simulink model "VCU_CS75_9_30"  (R2014a)
settings: Solver=FixedStepDiscrete  StartTime=0.0  StopTime=25  FixedStep=0.0005  RelTol=1e-3
undefined symbols (not defined in the file or in its folder): APAStatus_2D4, ecucoder_acal, I_SW01_L, LDW, ST_comd, TX2D4
libraries: simulink x881, ec5744lib x37
(part 13 of 30)

== system VCU_CS75_9_30/长安CS75底盘程序，20ms一次/BSW_Input/DBC转化的messages（存底）/ReceiveMessages12/HU_LASSetting_0x541/HU_LDWShakeLev_Sub ==
  In1 : Inport
  Out1 : Outport
  wires:
  In1/1 -> Out1/1

== system VCU_CS75_9_30/长安CS75底盘程序，20ms一次/BSW_Input/DBC转化的messages（存底）/ReceiveMessages12/HU_LASSetting_0x541/HU_LdwSensitivity_Sub ==
  In1 : Inport
  Out1 : Outport
  wires:
  In1/1 -> Out1/1

== system VCU_CS75_9_30/长安CS75底盘程序，20ms一次/BSW_Input/DBC转化的messages（存底）/ReceiveMessages12/HU_LASSetting_0x541/HU_LockCtrlEnable_Sub ==
  In1 : Inport
  Out1 : Outport
  wires:
  In1/1 -> Out1/1

== system VCU_CS75_9_30/长安CS75底盘程序，20ms一次/BSW_Input/DBC转化的messages（存底）/ReceiveMessages12/HU_LASSetting_0x541/HU_ObstacleSafeDistanceSet_Sub ==
  In1 : Inport
  Out1 : Outport
  wires:
  In1/1 -> Out1/1

== system VCU_CS75_9_30/长安CS75底盘程序，20ms一次/BSW_Input/DBC转化的messages（存底）/ReceiveMessages12/HU_LASSetting_0x541/HU_OverspeedSoundWarEnable_Sub ==
  In1 : Inport
  Out1 : Outport
  wires:
  In1/1 -> Out1/1

== system VCU_CS75_9_30/长安CS75底盘程序，20ms一次/BSW_Input/DBC转化的messages（存底）/ReceiveMessages12/HU_LASSetting_0x541/HU_OverspeedWarningEnable_Sub ==
  In1 : Inport
  Out1 : Outport
  wires:
  In1/1 -> Out1/1

== system VCU_CS75_9_30/长安CS75底盘程序，20ms一次/BSW_Input/DBC转化的messages（存底）/ReceiveMessages12/HU_LASSetting_0x541/HU_OverspeedWarningOffset_Sub ==
  In1 : Inport
  Out1 : Outport
  wires:
  In1/1 -> Out1/1

== system VCU_CS75_9_30/长安CS75底盘程序，20ms一次/BSW_Input/DBC转化的messages（存底）/ReceiveMessages12/HU_LASSetting_0x541/HU_ParkingConfirm_Sub ==
  In1 : Inport
  Out1 : Outport
  wires:
  In1/1 -> Out1/1

== system VCU_CS75_9_30/长安CS75底盘程序，20ms一次/BSW_Input/DBC转化的messages（存底）/ReceiveMessages12/HU_LASSetting_0x541/HU_ParkingResume_Sub ==
  In1 : Inport
  Out1 : Outport
  wires:
  In1/1 -> Out1/1

== system VCU_CS75_9_30/长安CS75底盘程序，20ms一次/BSW_Input/DBC转化的messages（存底）/ReceiveMessages12/HU_LASSetting_0x541/HU_RCWEnable_Sub ==
  In1 : Inport
  Out1 : Outport
  wires:
  In1/1 -> Out1/1

== system VCU_CS75_9_30/长安CS75底盘程序，20ms一次/BSW_Input/DBC转化的messages（存底）/ReceiveMessages12/HU_LASSetting_0x541/HU_RCWSoundEnable_Sub ==
  In1 : Inport
  Out1 : Outport
  wires:
  In1/1 -> Out1/1

== system VCU_CS75_9_30/长安CS75底盘程序，20ms一次/BSW_Input/DBC转化的messages（存底）/ReceiveMessages12/HU_LASSetting_0x541/HU_RemoteDistanceSet_Sub ==
  In1 : Inport
  Out1 : Outport
  wires:
  In1/1 -> Out1/1

== system VCU_CS75_9_30/长安CS75底盘程序，20ms一次/BSW_Input/DBC转化的messages（存底）/ReceiveMessages12/HU_LASSetting_0x541/HU_SEWEnable_Sub ==
  In1 : Inport
  Out1 : Outport
  wires:
  In1/1 -> Out1/1

== system VCU_CS75_9_30/长安CS75底盘程序，20ms一次/BSW_Input/DBC转化的messages（存底）/ReceiveMessages12/HU_LASSetting_0x541/HU_SLASwitch_Sub ==
  In1 : Inport
  Out1 : Outport
  wires:
  In1/1 -> Out1/1

== system VCU_CS75_9_30/长安CS75底盘程序，20ms一次/BSW_Input/DBC转化的messages（存底）/ReceiveMessages12/HU_LASSetting_0x541/HU_Uls_BSD_Activation_Sub ==
  In1 : Inport
  Out1 : Outport
  wires:
  In1/1 -> Out1/1

== system VCU_CS75_9_30/长安CS75底盘程序，20ms一次/BSW_Input/DBC转化的messages（存底）/ReceiveMessages12/HU_LASSetting_0x541/HU_Uls_FKP_Activation_Sub ==
  In1 : Inport
  Out1 : Outport
  wires:
  In1/1 -> Out1/1

== system VCU_CS75_9_30/长安CS75底盘程序，20ms一次/BSW_Input/DBC转化的messages（存底）/ReceiveMessages13/SAS_108/SAS_CRCCheck_Sub ==
  In1 : Inport
  Out1 : Outport
  wires:
  In1/1 -> Out1/1

== system VCU_CS75_9_30/长安CS75底盘程序，20ms一次/BSW_Input/DBC转化的messages（存底）/ReceiveMessages13/SAS_108/SAS_Calibrated_Sub ==
  In1 : Inport
  Out1 : Outport
  wires:
  In1/1 -> Out1/1

== system VCU_CS75_9_30/长安CS75底盘程序，20ms一次/BSW_Input/DBC转化的messages（存底）/ReceiveMessages13/SAS_108/SAS_RollingCounter_Sub ==
  In1 : Inport
  Out1 : Outport
  wires:
  In1/1 -> Out1/1

== system VCU_CS75_9_30/长安CS75底盘程序，20ms一次/BSW_Input/DBC转化的messages（存底）/ReceiveMessages13/SAS_108/SAS_SASFailure_Sub ==
  In1 : Inport
  Out1 : Outport
  wires:
  In1/1 -> Out1/1

== system VCU_CS75_9_30/长安CS75底盘程序，20ms一次/BSW_Input/DBC转化的messages（存底）/ReceiveMessages13/SAS_108/SAS_SteeringAngleSpeed_Sub ==
  In1 : Inport
  Out1 : Outport
  wires:
  In1/1 -> Out1/1

== system VCU_CS75_9_30/长安CS75底盘程序，20ms一次/BSW_Input/DBC转化的messages（存底）/ReceiveMessages13/SAS_108/SAS_SteeringAngleValid_Sub ==
  In1 : Inport
  Out1 : Outport
  wires:
  In1/1 -> Out1/1

== system VCU_CS75_9_30/长安CS75底盘程序，20ms一次/BSW_Input/DBC转化的messages（存底）/ReceiveMessages13/SAS_108/SAS_SteeringAngle_Sub ==
  In1 : Inport
  Out1 : Outport
  wires:
  In1/1 -> Out1/1

== system VCU_CS75_9_30/长安CS75底盘程序，20ms一次/BSW_Input/DBC转化的messages（存底）/ReceiveMessages14/SCM_3B8/SCM_ACCCancel_Sub ==
  In1 : Inport
  Out1 : Outport
  wires:
  In1/1 -> Out1/1

== system VCU_CS75_9_30/长安CS75底盘程序，20ms一次/BSW_Input/DBC转化的messages（存底）/ReceiveMessages14/SCM_3B8/SCM_ACCOn_Sub ==
  In1 : Inport
  Out1 : Outport
  wires:
  In1/1 -> Out1/1

== system VCU_CS75_9_30/长安CS75底盘程序，20ms一次/BSW_Input/DBC转化的messages（存底）/ReceiveMessages14/SCM_3B8/SCM_IACCOn_Sub ==
  In1 : Inport
  Out1 : Outport
  wires:
  In1/1 -> Out1/1

== system VCU_CS75_9_30/长安CS75底盘程序，20ms一次/BSW_Input/DBC转化的messages（存底）/ReceiveMessages14/SCM_3B8/SCM_Resume_Sub ==
  In1 : Inport
  Out1 : Outport
  wires:
  In1/1 -> Out1/1

== system VCU_CS75_9_30/长安CS75底盘程序，20ms一次/BSW_Input/DBC转化的messages（存底）/ReceiveMessages14/SCM_3B8/SCM_Speeddecrease_Sub ==
  In1 : Inport
  Out1 : Outport
  wires:
  In1/1 -> Out1/1

== system VCU_CS75_9_30/长安CS75底盘程序，20ms一次/BSW_Input/DBC转化的messages（存底）/ReceiveMessages14/SCM_3B8/SCM_TimeGap_Sub ==
  In1 : Inport
  Out1 : Outport
  wires:
  In1/1 -> Out1/1

== system VCU_CS75_9_30/长安CS75底盘程序，20ms一次/BSW_Input/DBC转化的messages（存底）/ReceiveMessages15/SRS_005/SRS_DriverBuckleSwitchStatus_Sub ==
  In1 : Inport
  Out1 : Outport
  wires:
  In1/1 -> Out1/1

== system VCU_CS75_9_30/长安CS75底盘程序，20ms一次/BSW_Input/DBC转化的messages（存底）/ReceiveMessages15/SRS_005/SRS_RollingCounter_Sub ==
  In1 : Inport
  Out1 : Outport
  wires:
  In1/1 -> Out1/1

== system VCU_CS75_9_30/长安CS75底盘程序，20ms一次/BSW_Input/DBC转化的messages（存底）/ReceiveMessages16/TCU_286/TCU_ActualGearValid_Sub ==
  In1 : Inport
  Out1 : Outport
  wires:
  In1/1 -> Out1/1

== system VCU_CS75_9_30/长安CS75底盘程序，20ms一次/BSW_Input/DBC转化的messages（存底）/ReceiveMessages16/TCU_286/TCU_ActualGear_Sub ==
  In1 : Inport
  Out1 : Outport
  wires:
  In1/1 -> Out1/1

== system VCU_CS75_9_30/长安CS75底盘程序，20ms一次/BSW_Input/DBC转化的messages（存底）/ReceiveMessages16/TCU_286/TCU_GearShiftPosition_Sub ==
  In1 : Inport
  Out1 : Outport
  wires:
  In1/1 -> Out1/1

== system VCU_CS75_9_30/长安CS75底盘程序，20ms一次/BSW_Input/DBC转化的messages（存底）/ReceiveMessages16/TCU_286/TCU_ShiftPositionValid_Sub ==
  In1 : Inport
  Out1 : Outport
  wires:
  In1/1 -> Out1/1

== system VCU_CS75_9_30/长安CS75底盘程序，20ms一次/BSW_Input/DBC转化的messages（存底）/ReceiveMessages17/BCM_288/BCM_BuzzerWarningMode_Sub ==
  In1 : Inport
  Out1 : Outport
  wires:
  In1/1 -> Out1/1

== system VCU_CS75_9_30/长安CS75底盘程序，20ms一次/BSW_Input/DBC转化的messages（存底）/ReceiveMessages17/BCM_288/BCM_DriverDoorLockStatus_Sub ==
  In1 : Inport
  Out1 : Outport
  wires:
  In1/1 -> Out1/1

== system VCU_CS75_9_30/长安CS75底盘程序，20ms一次/BSW_Input/DBC转化的messages（存底）/ReceiveMessages17/BCM_288/BCM_DriverDoorStatus_Sub ==
  In1 : Inport
  Out1 : Outport
  wires:
  In1/1 -> Out1/1

== system VCU_CS75_9_30/长安CS75底盘程序，20ms一次/BSW_Input/DBC转化的messages（存底）/ReceiveMessages17/BCM_288/BCM_FrontWashStatus_Sub ==
  In1 : Inport
  Out1 : Outport
  wires:
  In1/1 -> Out1/1

== system VCU_CS75_9_30/长安CS75底盘程序，20ms一次/BSW_Input/DBC转化的messages（存底）/ReceiveMessages17/BCM_288/BCM_FrontWiperStatus_Sub ==
  In1 : Inport
  Out1 : Outport
  wires:
  In1/1 -> Out1/1

== system VCU_CS75_9_30/长安CS75底盘程序，20ms一次/BSW_Input/DBC转化的messages（存底）/ReceiveMessages17/BCM_288/BCM_HoodStatus_Sub ==
  In1 : Inport
  Out1 : Outport
  wires:
  In1/1 -> Out1/1

== system VCU_CS75_9_30/长安CS75底盘程序，20ms一次/BSW_Input/DBC转化的messages（存底）/ReceiveMessages17/BCM_288/BCM_LatchOverheatProtect_Sub ==
  In1 : Inport
  Out1 : Outport
  wires:
  In1/1 -> Out1/1

== system VCU_CS75_9_30/长安CS75底盘程序，20ms一次/BSW_Input/DBC转化的messages（存底）/ReceiveMessages17/BCM_288/BCM_LeftRearDoorStatus_Sub ==
  In1 : Inport
  Out1 : Outport
  wires:
  In1/1 -> Out1/1

== system VCU_CS75_9_30/长安CS75底盘程序，20ms一次/BSW_Input/DBC转化的messages（存底）/ReceiveMessages17/BCM_288/BCM_PassengerDoorLockStatus_Sub ==
  In1 : Inport
  Out1 : Outport
  wires:
  In1/1 -> Out1/1

== system VCU_CS75_9_30/长安CS75底盘程序，20ms一次/BSW_Input/DBC转化的messages（存底）/ReceiveMessages17/BCM_288/BCM_PassengerDoorStatus_Sub ==
  In1 : Inport
  Out1 : Outport
  wires:
  In1/1 -> Out1/1

== system VCU_CS75_9_30/长安CS75底盘程序，20ms一次/BSW_Input/DBC转化的messages（存底）/ReceiveMessages17/BCM_288/BCM_PowerStatusFeedback_Sub ==
  In1 : Inport
  Out1 : Outport
  wires:
  In1/1 -> Out1/1

== system VCU_CS75_9_30/长安CS75底盘程序，20ms一次/BSW_Input/DBC转化的messages（存底）/ReceiveMessages17/BCM_288/BCM_RearWiperStatus_Sub ==
  In1 : Inport
  Out1 : Outport
  wires:
  In1/1 -> Out1/1

== system VCU_CS75_9_30/长安CS75底盘程序，20ms一次/BSW_Input/DBC转化的messages（存底）/ReceiveMessages17/BCM_288/BCM_ReversePosition_Sub ==
  In1 : Inport
  Out1 : Outport
  wires:
  In1/1 -> Out1/1

== system VCU_CS75_9_30/长安CS75底盘程序，20ms一次/BSW_Input/DBC转化的messages（存底）/ReceiveMessages17/BCM_288/BCM_RightRearDoorStatus_Sub ==
  In1 : Inport
  Out1 : Outport
  wires:
  In1/1 -> Out1/1

== system VCU_CS75_9_30/长安CS75底盘程序，20ms一次/BSW_Input/DBC转化的messages（存底）/ReceiveMessages17/BCM_288/BCM_SystemFailureFlag_Sub ==
  In1 : Inport
  Out1 : Outport
  wires:
  In1/1 -> Out1/1

== system VCU_CS75_9_30/长安CS75底盘程序，20ms一次/BSW_Input/DBC转化的messages（存底）/ReceiveMessages17/BCM_288/BCM_TrunkDoorStatus_Sub ==
  In1 : Inport
  Out1 : Outport
  wires:
  In1/1 -> Out1/1

== system VCU_CS75_9_30/长安CS75底盘程序，20ms一次/BSW_Input/DBC转化的messages（存底）/ReceiveMessages17/BCM_288/BCM_TurnIndicatorLeft_Sub ==
  In1 : Inport
  Out1 : Outport
  wires:
  In1/1 -> Out1/1

== system VCU_CS75_9_30/长安CS75底盘程序，20ms一次/BSW_Input/DBC转化的messages（存底）/ReceiveMessages17/BCM_288/BCM_TurnIndicatorRight_Sub ==
  In1 : Inport
  Out1 : Outport
  wires:
  In1/1 -> Out1/1

== system VCU_CS75_9_30/长安CS75底盘程序，20ms一次/BSW_Input/DBC转化的messages（存底）/ReceiveMessages17/BCM_288/BCM_TurnLightSwitchSts_Sub ==
  In1 : Inport
  Out1 : Outport
  wires:
  In1/1 -> Out1/1

== system VCU_CS75_9_30/长安CS75底盘程序，20ms一次/BSW_Input/DBC转化的messages（存底）/ReceiveMessages17/BCM_288/BCM_emergencylightstatus_Sub ==
  In1 : Inport
  Out1 : Outport
  wires:
  In1/1 -> Out1/1

== system VCU_CS75_9_30/长安CS75底盘程序，20ms一次/BSW_Input/DBC转化的messages（存底）/ReceiveMessages18/BCM_328/LCM_DRLSts_Sub ==
  In1 : Inport
  Out1 : Outport
  wires:
  In1/1 -> Out1/1

== system VCU_CS75_9_30/长安CS75底盘程序，20ms一次/BSW_Input/DBC转化的messages（存底）/ReceiveMessages18/BCM_328/LCM_DriveMode_Sub ==
  In1 : Inport
  Out1 : Outport
  wires:
  In1/1 -> Out1/1

== system VCU_CS75_9_30/长安CS75底盘程序，20ms一次/BSW_Input/DBC转化的messages（存底）/ReceiveMessages18/BCM_328/LCM_LASSwitch_Sub ==
  In1 : Inport
  Out1 : Outport
  wires:
  In1/1 -> Out1/1

== system VCU_CS75_9_30/长安CS75底盘程序，20ms一次/BSW_Input/DBC转化的messages（存底）/ReceiveMessages18/BCM_328/LCM_RearLeftTuningLightFaultSts_Sub ==
  In1 : Inport
  Out1 : Outport
  wires:
  In1/1 -> Out1/1

== system VCU_CS75_9_30/长安CS75底盘程序，20ms一次/BSW_Input/DBC转化的messages（存底）/ReceiveMessages18/BCM_328/LCM_RearRightTuningLightFaultSts_Sub ==
  In1 : Inport
  Out1 : Outport
  wires:
  In1/1 -> Out1/1

== system VCU_CS75_9_30/长安CS75底盘程序，20ms一次/BSW_Input/DBC转化的messages（存底）/ReceiveMessages18/BCM_328/LCM_ReverseLightSts_Sub ==
  In1 : Inport
  Out1 : Outport
  wires:
  In1/1 -> Out1/1

== system VCU_CS75_9_30/长安CS75底盘程序，20ms一次/BSW_Input/DBC转化的messages（存底）/ReceiveMessages19/BCM_348/BCM_DriveMode_Sub ==
  In1 : Inport
  Out1 : Outport
  wires:
  In1/1 -> Out1/1

== system VCU_CS75_9_30/长安CS75底盘程序，20ms一次/BSW_Input/DBC转化的messages（存底）/ReceiveMessages19/BCM_348/BCM_LockSignal_Sub ==
  In1 : Inport
  Out1 : Outport
  wires:
  In1/1 -> Out1/1

== system VCU_CS75_9_30/长安CS75底盘程序，20ms一次/BSW_Input/DBC转化的messages（存底）/ReceiveMessages19/BCM_348/BCM_UnlockSignal_Sub ==
  In1 : Inport
  Out1 : Outport
  wires:
  In1/1 -> Out1/1

== system VCU_CS75_9_30/长安CS75底盘程序，20ms一次/BSW_Input/DBC转化的messages（存底）/ReceiveMessages2/EMS_265/EMS_EngineStatus_Sub ==
  In1 : Inport
  Out1 : Outport
  wires:
  In1/1 -> Out1/1

== system VCU_CS75_9_30/长安CS75底盘程序，20ms一次/BSW_Input/DBC转化的messages（存底）/ReceiveMessages2/EMS_265/EMS_FullLoadIndicatedTorq_Sub ==
  In1 : Inport
  Out1 : Outport
  wires:
  In1/1 -> Out1/1

== system VCU_CS75_9_30/长安CS75底盘程序，20ms一次/BSW_Input/DBC转化的messages（存底）/ReceiveMessages2/EMS_265/EMS_RollingCounter_id265_Sub ==
  In1 : Inport
  Out1 : Outport
  wires:
  In1/1 -> Out1/1

== system VCU_CS75_9_30/长安CS75底盘程序，20ms一次/BSW_Input/DBC转化的messages（存底）/ReceiveMessages2/EMS_265/EMS_TorqueConstant_Sub ==
  In1 : Inport
  Out1 : Outport
  wires:
  In1/1 -> Out1/1

== system VCU_CS75_9_30/长安CS75底盘程序，20ms一次/BSW_Input/DBC转化的messages（存底）/ReceiveMessages20/BCM_3DF/BCM_AmbientLightColorFeedback_Sub ==
  In1 : Inport
  Out1 : Outport
  wires:
  In1/1 -> Out1/1

== system VCU_CS75_9_30/长安CS75底盘程序，20ms一次/BSW_Input/DBC转化的messages（存底）/ReceiveMessages20/BCM_3DF/BCM_CRC_Checksum_Sub ==
  In1 : Inport
  Out1 : Outport
  wires:
  In1/1 -> Out1/1

== system VCU_CS75_9_30/长安CS75底盘程序，20ms一次/BSW_Input/DBC转化的messages（存底）/ReceiveMessages20/BCM_3DF/BCM_DriveModeFeedback_Sub ==
  In1 : Inport
  Out1 : Outport
  wires:
  In1/1 -> Out1/1

== system VCU_CS75_9_30/长安CS75底盘程序，20ms一次/BSW_Input/DBC转化的messages（存底）/ReceiveMessages20/BCM_3DF/BCM_DriveModeStatus_Sub ==
  In1 : Inport
  Out1 : Outport
  wires:
  In1/1 -> Out1/1

== system VCU_CS75_9_30/长安CS75底盘程序，20ms一次/BSW_Input/DBC转化的messages（存底）/ReceiveMessages20/BCM_3DF/BCM_DriveMode_Sub ==
  In1 : Inport
  Out1 : Outport
  wires:
  In1/1 -> Out1/1

== system VCU_CS75_9_30/长安CS75底盘程序，20ms一次/BSW_Input/DBC转化的messages（存底）/ReceiveMessages20/BCM_3DF/BCM_EPSTorqueModeFeedback_Sub ==
  In1 : Inport
  Out1 : Outport
  wires:
  In1/1 -> Out1/1

== system VCU_CS75_9_30/长安CS75底盘程序，20ms一次/BSW_Input/DBC转化的messages（存底）/ReceiveMessages20/BCM_3DF/BCM_EPSTorqueMode_Sub ==
  In1 : Inport
  Out1 : Outport
  wires:
  In1/1 -> Out1/1

== system VCU_CS75_9_30/长安CS75底盘程序，20ms一次/BSW_Input/DBC转化的messages（存底）/ReceiveMessages20/BCM_3DF/BCM_RollingCounter_Sub ==
  In1 : Inport
  Out1 : Outport
  wires:
  In1/1 -> Out1/1

== system VCU_CS75_9_30/长安CS75底盘程序，20ms一次/BSW_Input/DBC转化的messages（存底）/ReceiveMessages21/GW_20B/EMS_BrakePedalStatus_Sub ==
  In1 : Inport
  Out1 : Outport
  wires:
  In1/1 -> Out1/1

== system VCU_CS75_9_30/长安CS75底盘程序，20ms一次/BSW_Input/DBC转化的messages（存底）/ReceiveMessages21/GW_20B/EMS_EngineStartupEnd_Sub ==
  In1 : Inport
  Out1 : Outport
  wires:
  In1/1 -> Out1/1

== system VCU_CS75_9_30/长安CS75底盘程序，20ms一次/BSW_Input/DBC转化的messages（存底）/ReceiveMessages21/GW_20B/EMS_EngineStatus_Sub ==
  In1 : Inport
  Out1 : Outport
  wires:
  In1/1 -> Out1/1

== system VCU_CS75_9_30/长安CS75底盘程序，20ms一次/BSW_Input/DBC转化的messages（存底）/ReceiveMessages21/GW_20B/EPB_BrakeLightOnRequest_Sub ==
  In1 : Inport
  Out1 : Outport
  wires:
  In1/1 -> Out1/1

== system VCU_CS75_9_30/长安CS75底盘程序，20ms一次/BSW_Input/DBC转化的messages（存底）/ReceiveMessages21/GW_20B/EPB_Status_Sub ==
  In1 : Inport
  Out1 : Outport
  wires:
  In1/1 -> Out1/1

== system VCU_CS75_9_30/长安CS75底盘程序，20ms一次/BSW_Input/DBC转化的messages（存底）/ReceiveMessages21/GW_20B/SAS_SteeringAngleValid_Sub ==
  In1 : Inport
  Out1 : Outport
  wires:
  In1/1 -> Out1/1

== system VCU_CS75_9_30/长安CS75底盘程序，20ms一次/BSW_Input/DBC转化的messages（存底）/ReceiveMessages21/GW_20B/SAS_SteeringAngle_Sub ==
  In1 : Inport
  Out1 : Outport
  wires:
  In1/1 -> Out1/1

== system VCU_CS75_9_30/长安CS75底盘程序，20ms一次/BSW_Input/DBC转化的messages（存底）/ReceiveMessages21/GW_20B/TCU_GearShiftPositon_Sub ==
  In1 : Inport
  Out1 : Outport
  wires:
  In1/1 -> Out1/1

== system VCU_CS75_9_30/长安CS75底盘程序，20ms一次/BSW_Input/DBC转化的messages（存底）/ReceiveMessages21/GW_20B/TCU_ShiftPostionValid_Sub ==
  In1 : Inport
  Out1 : Outport
  wires:
  In1/1 -> Out1/1

== system VCU_CS75_9_30/长安CS75底盘程序，20ms一次/BSW_Input/DBC转化的messages（存底）/ReceiveMessages22/GW_332/EMS_EngineSpeed_Sub ==
  In1 : Inport
  Out1 : Outport
  wires:
  In1/1 -> Out1/1

== system VCU_CS75_9_30/长安CS75底盘程序，20ms一次/BSW_Input/DBC转化的messages（存底）/ReceiveMessages22/GW_332/SAS_SASFailure_Sub ==
  In1 : Inport
  Out1 : Outport
  wires:
  In1/1 -> Out1/1

== system VCU_CS75_9_30/长安CS75底盘程序，20ms一次/BSW_Input/DBC转化的messages（存底）/ReceiveMessages22/GW_332/SRS_DriverBuckleSwitchStatus_Sub ==
  In1 : Inport
  Out1 : Outport
  wires:
  In1/1 -> Out1/1

== system VCU_CS75_9_30/长安CS75底盘程序，20ms一次/BSW_Input/DBC转化的messages（存底）/ReceiveMessages22/GW_332/SRS_PassengerBuckleSwitchStatus_Sub ==
  In1 : Inport
  Out1 : Outport
  wires:
  In1/1 -> Out1/1

== system VCU_CS75_9_30/长安CS75底盘程序，20ms一次/BSW_Input/DBC转化的messages（存底）/ReceiveMessages23/GW_308/IP_TotalOdometer_Sub ==
  In1 : Inport
  Out1 : Outport
  wires:
  In1/1 -> Out1/1

== system VCU_CS75_9_30/长安CS75底盘程序，20ms一次/BSW_Input/DBC转化的messages（存底）/ReceiveMessages24/GW_376/EMS_ConditionIdle_Sub ==
  In1 : Inport
  Out1 : Outport
  wires:
  In1/1 -> Out1/1

== system VCU_CS75_9_30/长安CS75底盘程序，20ms一次/BSW_Input/DBC转化的messages（存底）/ReceiveMessages24/GW_376/EMS_EngineFuelCutOff_Sub ==
  In1 : Inport
  Out1 : Outport
  wires:
  In1/1 -> Out1/1

== system VCU_CS75_9_30/长安CS75底盘程序，20ms一次/BSW_Input/DBC转化的messages（存底）/ReceiveMessages24/GW_376/EMS_FrictionalTorq_Sub ==
  In1 : Inport
  Out1 : Outport
  wires:
  In1/1 -> Out1/1

== system VCU_CS75_9_30/长安CS75底盘程序，20ms一次/BSW_Input/DBC转化的messages（存底）/ReceiveMessages24/GW_376/EMS_TorqueConstant_Sub ==
  In1 : Inport
  Out1 : Outport
  wires:
  In1/1 -> Out1/1

== system VCU_CS75_9_30/长安CS75底盘程序，20ms一次/BSW_Input/DBC转化的messages（存底）/ReceiveMessages25/GW_3A2/ACC_ACCMode_Sub ==
  In1 : Inport
  Out1 : Outport
  wires:
  In1/1 -> Out1/1

== system VCU_CS75_9_30/长安CS75底盘程序，20ms一次/BSW_Input/DBC转化的messages（存底）/ReceiveMessages25/GW_3A2/EMS_RemindGear_Sub ==
  In1 : Inport
  Out1 : Outport
  wires:
  In1/1 -> Out1/1

== system VCU_CS75_9_30/长安CS75底盘程序，20ms一次/BSW_Input/DBC转化的messages（存底）/ReceiveMessages25/GW_3A2/EMS_RemindShiftGear_Sub ==
  In1 : Inport
  Out1 : Outport
  wires:
  In1/1 -> Out1/1

== system VCU_CS75_9_30/长安CS75底盘程序，20ms一次/BSW_Input/DBC转化的messages（存底）/ReceiveMessages25/GW_3A2/EPB_FunctionLamp_Sub ==
  In1 : Inport
  Out1 : Outport
  wires:
  In1/1 -> Out1/1

== system VCU_CS75_9_30/长安CS75底盘程序，20ms一次/BSW_Input/DBC转化的messages（存底）/ReceiveMessages25/GW_3A2/EPB_SwitchPositionValid_Sub ==
  In1 : Inport
  Out1 : Outport
  wires:
  In1/1 -> Out1/1

== system VCU_CS75_9_30/长安CS75底盘程序，20ms一次/BSW_Input/DBC转化的messages（存底）/ReceiveMessages25/GW_3A2/EPB_SwitchPosition_Sub ==
  In1 : Inport
  Out1 : Outport
  wires:
  In1/1 -> Out1/1

== system VCU_CS75_9_30/长安CS75底盘程序，20ms一次/BSW_Input/DBC转化的messages（存底）/ReceiveMessages25/GW_3A2/EPB_TextDisplay_Sub ==
  In1 : Inport
  Out1 : Outport
  wires:
  In1/1 -> Out1/1

== system VCU_CS75_9_30/长安CS75底盘程序，20ms一次/BSW_Input/DBC转化的messages（存底）/ReceiveMessages25/GW_3A2/EPS_EPSFailed_Sub ==
  In1 : Inport
  Out1 : Outport
  wires:
  In1/1 -> Out1/1

== system VCU_CS75_9_30/长安CS75底盘程序，20ms一次/BSW_Input/DBC转化的messages（存底）/ReceiveMessages25/GW_3A2/EPS_TorqueAssistMode_Sub ==
  In1 : Inport
  Out1 : Outport
  wires:
  In1/1 -> Out1/1

== system VCU_CS75_9_30/长安CS75底盘程序，20ms一次/BSW_Input/DBC转化的messages（存底）/ReceiveMessages25/GW_3A2/ESP_AutoHoldActive_Sub ==
  In1 : Inport
  Out1 : Outport
  wires:
  In1/1 -> Out1/1

== system VCU_CS75_9_30/长安CS75底盘程序，20ms一次/BSW_Input/DBC转化的messages（存底）/ReceiveMessages25/GW_3A2/ESP_AutoHoldAvailable_Sub ==
  In1 : Inport
  Out1 : Outport
  wires:
  In1/1 -> Out1/1

== system VCU_CS75_9_30/长安CS75底盘程序，20ms一次/BSW_Input/DBC转化的messages（存底）/ReceiveMessages25/GW_3A2/ESP_EBDFailStatus_Sub ==
  In1 : Inport
  Out1 : Outport
  wires:
  In1/1 -> Out1/1

== system VCU_CS75_9_30/长安CS75底盘程序，20ms一次/BSW_Input/DBC转化的messages（存底）/ReceiveMessages25/GW_3A2/ESP_ESPActiveStatus_Sub ==
  In1 : Inport
  Out1 : Outport
  wires:
  In1/1 -> Out1/1

== system VCU_CS75_9_30/长安CS75底盘程序，20ms一次/BSW_Input/DBC转化的messages（存底）/ReceiveMessages25/GW_3A2/ESP_ESPFunctionStatus_Sub ==
  In1 : Inport
  Out1 : Outport
  wires:
  In1/1 -> Out1/1

== system VCU_CS75_9_30/长安CS75底盘程序，20ms一次/BSW_Input/DBC转化的messages（存底）/ReceiveMessages25/GW_3A2/ESP_HBBFunctionStatus_Sub ==
  In1 : Inport
  Out1 : Outport
  wires:
  In1/1 -> Out1/1

== system VCU_CS75_9_30/长安CS75底盘程序，20ms一次/BSW_Input/DBC转化的messages（存底）/ReceiveMessages25/GW_3A2/ESP_HDC_STATUS_Sub ==
  In1 : Inport
  Out1 : Outport
  wires:
  In1/1 -> Out1/1

== system VCU_CS75_9_30/长安CS75底盘程序，20ms一次/BSW_Input/DBC转化的messages（存底）/ReceiveMessages25/GW_3A2/ESP_HHC_Active_Sub ==
  In1 : Inport
  Out1 : Outport
  wires:
  In1/1 -> Out1/1

== system VCU_CS75_9_30/长安CS75底盘程序，20ms一次/BSW_Input/DBC转化的messages（存底）/ReceiveMessages25/GW_3A2/ESP_HHC_Available_Sub ==
  In1 : Inport
  Out1 : Outport
  wires:
  In1/1 -> Out1/1

== system VCU_CS75_9_30/长安CS75底盘程序，20ms一次/BSW_Input/DBC转化的messages（存底）/ReceiveMessages25/GW_3A2/SRS_LeftRearBuckleSwitchSts_Sub ==
  In1 : Inport
  Out1 : Outport
  wires:
  In1/1 -> Out1/1

== system VCU_CS75_9_30/长安CS75底盘程序，20ms一次/BSW_Input/DBC转化的messages（存底）/ReceiveMessages25/GW_3A2/SRS_MiddleRearBuckleSwitchSts_Sub ==
  In1 : Inport
  Out1 : Outport
  wires:
  In1/1 -> Out1/1

== system VCU_CS75_9_30/长安CS75底盘程序，20ms一次/BSW_Input/DBC转化的messages（存底）/ReceiveMessages25/GW_3A2/SRS_RightRearBuckleSwitchSts_Sub ==
  In1 : Inport
  Out1 : Outport
  wires:
  In1/1 -> Out1/1

== system VCU_CS75_9_30/长安CS75底盘程序，20ms一次/BSW_Input/DBC转化的messages（存底）/ReceiveMessages25/GW_3A2/TCU_FailureLamp_Sub ==
  In1 : Inport
  Out1 : Outport
  wires:
  In1/1 -> Out1/1

== system VCU_CS75_9_30/长安CS75底盘程序，20ms一次/BSW_Input/DBC转化的messages（存底）/ReceiveMessages25/GW_3A2/TCU_GearForDisplay_Sub ==
  In1 : Inport
  Out1 : Outport
  wires:
  In1/1 -> Out1/1

== system VCU_CS75_9_30/长安CS75底盘程序，20ms一次/BSW_Input/DBC转化的messages（存底）/ReceiveMessages25/GW_3A2/TCU_GearIndication_Sub ==
  In1 : Inport
  Out1 : Outport
  wires:
  In1/1 -> Out1/1

== system VCU_CS75_9_30/长安CS75底盘程序，20ms一次/BSW_Input/DBC转化的messages（存底）/ReceiveMessages25/GW_3A2/TCU_PWRLamp_Sub ==
  In1 : Inport
  Out1 : Outport
  wires:
  In1/1 -> Out1/1

== system VCU_CS75_9_30/长安CS75底盘程序，20ms一次/BSW_Input/DBC转化的messages（存底）/ReceiveMessages25/GW_3A2/TCU_ReqTranTempWarning_Sub ==
  In1 : Inport
  Out1 : Outport
  wires:
  In1/1 -> Out1/1

== system VCU_CS75_9_30/长安CS75底盘程序，20ms一次/BSW_Input/DBC转化的messages（存底）/ReceiveMessages25/GW_3A2/TCU_WNTLamp_Sub ==
  In1 : Inport
  Out1 : Outport
  wires:
  In1/1 -> Out1/1

== system VCU_CS75_9_30/长安CS75底盘程序，20ms一次/BSW_Input/DBC转化的messages（存底）/ReceiveMessages26/GW_567/HU_Byroad_Sub ==
  In1 : Inport
  Out1 : Outport
  wires:
  In1/1 -> Out1/1

== system VCU_CS75_9_30/长安CS75底盘程序，20ms一次/BSW_Input/DBC转化的messages（存底）/ReceiveMessages26/GW_567/HU_EnterTunnelInfo_Sub ==
  In1 : Inport
  Out1 : Outport
  wires:
  In1/1 -> Out1/1

== system VCU_CS75_9_30/长安CS75底盘程序，20ms一次/BSW_Input/DBC转化的messages（存底）/ReceiveMessages26/GW_567/HU_NavGuiganceStatus_Sub ==
  In1 : Inport
  Out1 : Outport
  wires:
  In1/1 -> Out1/1

== system VCU_CS75_9_30/长安CS75底盘程序，20ms一次/BSW_Input/DBC转化的messages（存底）/ReceiveMessages26/GW_567/HU_TunnelDistance_Sub ==
  In1 : Inport
  Out1 : Outport
  wires:
  In1/1 -> Out1/1

== system VCU_CS75_9_30/长安CS75底盘程序，20ms一次/BSW_Input/DBC转化的messages（存底）/ReceiveMessages26/GW_567/HU_TunnelLength_Sub ==
  In1 : Inport
  Out1 : Outport
  wires:
  In1/1 -> Out1/1

== system VCU_CS75_9_30/长安CS75底盘程序，20ms一次/BSW_Input/DBC转化的messages（存底）/ReceiveMessages27/HU_GPS_500/GPSCurrentLocationValid_Sub ==
  In1 : Inport
  Out1 : Outport
  wires:
  In1/1 -> Out1/1

== system VCU_CS75_9_30/长安CS75底盘程序，20ms一次/BSW_Input/DBC转化的messages（存底）/ReceiveMessages28/LAS_36E/LAS_CheckSum_id36E_Sub ==
  In1 : Inport
  Out1 : Outport
  wires:
  In1/1 -> Out1/1

== system VCU_CS75_9_30/长安CS75底盘程序，20ms一次/BSW_Input/DBC转化的messages（存底）/ReceiveMessages28/LAS_36E/LAS_LaneEquationC1_Sub ==
  In1 : Inport
  Out1 : Outport
  wires:
  In1/1 -> Out1/1

== system VCU_CS75_9_30/长安CS75底盘程序，20ms一次/BSW_Input/DBC转化的messages（存底）/ReceiveMessages28/LAS_36E/LAS_LaneEquationC3_Sub ==
  In1 : Inport
  Out1 : Outport
  wires:
  In1/1 -> Out1/1

== system VCU_CS75_9_30/长安CS75底盘程序，20ms一次/BSW_Input/DBC转化的messages（存底）/ReceiveMessages28/LAS_36E/LAS_LaneEquationStatus_Sub ==
  In1 : Inport
  Out1 : Outport
  wires:
  In1/1 -> Out1/1

== system VCU_CS75_9_30/长安CS75底盘程序，20ms一次/BSW_Input/DBC转化的messages（存底）/ReceiveMessages28/LAS_36E/LAS_RoadCurvatureFar_Sub ==
  In1 : Inport
  Out1 : Outport
  wires:
  In1/1 -> Out1/1

== system VCU_CS75_9_30/长安CS75底盘程序，20ms一次/BSW_Input/DBC转化的messages（存底）/ReceiveMessages28/LAS_36E/LAS_RoadCurvatureNear_Sub ==
  In1 : Inport
  Out1 : Outport
  wires:
  In1/1 -> Out1/1

== system VCU_CS75_9_30/长安CS75底盘程序，20ms一次/BSW_Input/DBC转化的messages（存底）/ReceiveMessages28/LAS_36E/LAS_RollingCounter_id36E_Sub ==
  In1 : Inport
  Out1 : Outport
  wires:
  In1/1 -> Out1/1

== system VCU_CS75_9_30/长安CS75底盘程序，20ms一次/BSW_Input/DBC转化的messages（存底）/ReceiveMessages3/EMS_276/EMS_RealAccPedal_Sub ==
  In1 : Inport
  Out1 : Outport
  wires:
  In1/1 -> Out1/1

== system VCU_CS75_9_30/长安CS75底盘程序，20ms一次/BSW_Input/DBC转化的messages（存底）/ReceiveMessages4/EPB_256/EPB_Checksum_Sub ==
  In1 : Inport
  Out1 : Outport
  wires:
  In1/1 -> Out1/1

== system VCU_CS75_9_30/长安CS75底盘程序，20ms一次/BSW_Input/DBC转化的messages（存底）/ReceiveMessages4/EPB_256/EPB_FailStatus_Sub ==
  In1 : Inport
  Out1 : Outport
  wires:
  In1/1 -> Out1/1

== system VCU_CS75_9_30/长安CS75底盘程序，20ms一次/BSW_Input/DBC转化的messages（存底）/ReceiveMessages4/EPB_256/EPB_FailureLamp_Sub ==
  In1 : Inport
  Out1 : Outport
  wires:
  In1/1 -> Out1/1

== system VCU_CS75_9_30/长安CS75底盘程序，20ms一次/BSW_Input/DBC转化的messages（存底）/ReceiveMessages4/EPB_256/EPB_FunctionLamp_Sub ==
  In1 : Inport
  Out1 : Outport
  wires:
  In1/1 -> Out1/1

== system VCU_CS75_9_30/长安CS75底盘程序，20ms一次/BSW_Input/DBC转化的messages（存底）/ReceiveMessages4/EPB_256/EPB_RollingCounter_id256_Sub ==
  In1 : Inport
  Out1 : Outport
  wires:
  In1/1 -> Out1/1

== system VCU_CS75_9_30/长安CS75底盘程序，20ms一次/BSW_Input/DBC转化的messages（存底）/ReceiveMessages4/EPB_256/EPB_Status_Sub ==
  In1 : Inport
  Out1 : Outport
  wires:
  In1/1 -> Out1/1

== system VCU_CS75_9_30/长安CS75底盘程序，20ms一次/BSW_Input/DBC转化的messages（存底）/ReceiveMessages5/EPS_20A/EPS_APA_AbortFeedback_Sub ==
  In1 : Inport
  Out1 : Outport
  wires:
  In1/1 -> Out1/1

== system VCU_CS75_9_30/长安CS75底盘程序，20ms一次/BSW_Input/DBC转化的messages（存底）/ReceiveMessages5/EPS_20A/EPS_APA_ControlFeedback_Sub ==
  In1 : Inport
  Out1 : Outport
  wires:
  In1/1 -> Out1/1

== system VCU_CS75_9_30/长安CS75底盘程序，20ms一次/BSW_Input/DBC转化的messages（存底）/ReceiveMessages5/EPS_20A/EPS_APA_EpasFailed_Sub ==
  In1 : Inport
  Out1 : Outport
  wires:
  In1/1 -> Out1/1

== system VCU_CS75_9_30/长安CS75底盘程序，20ms一次/BSW_Input/DBC转化的messages（存底）/ReceiveMessages5/EPS_20A/EPS_Checksum_Sub ==
  In1 : Inport
  Out1 : Outport
  wires:
  In1/1 -> Out1/1

== system VCU_CS75_9_30/长安CS75底盘程序，20ms一次/BSW_Input/DBC转化的messages（存底）/ReceiveMessages5/EPS_20A/EPS_ConcussAvailabilityStatus_Sub ==
  In1 : Inport
  Out1 : Outport
  wires:
  In1/1 -> Out1/1

== system VCU_CS75_9_30/长安CS75底盘程序，20ms一次/BSW_Input/DBC转化的messages（存底）/ReceiveMessages5/EPS_20A/EPS_EPSFailed_Sub ==
  In1 : Inport
  Out1 : Outport
  wires:
  In1/1 -> Out1/1

== system VCU_CS75_9_30/长安CS75底盘程序，20ms一次/BSW_Input/DBC转化的messages（存底）/ReceiveMessages5/EPS_20A/EPS_RollingCounter_Sub ==
  In1 : Inport
  Out1 : Outport
  wires:
  In1/1 -> Out1/1

== system VCU_CS75_9_30/长安CS75底盘程序，20ms一次/BSW_Input/DBC转化的messages（存底）/ReceiveMessages5/EPS_20A/EPS_SteeringTorque_Sub ==
  In1 : Inport
  Out1 : Outport
  wires:
  In1/1 -> Out1/1

== system VCU_CS75_9_30/长安CS75底盘程序，20ms一次/BSW_Input/DBC转化的messages（存底）/ReceiveMessages5/EPS_20A/EPS_TorqueSensorStatus_Sub ==
  In1 : Inport
  Out1 : Outport
  wires:
  In1/1 -> Out1/1

== system VCU_CS75_9_30/长安CS75底盘程序，20ms一次/BSW_Input/DBC转化的messages（存底）/ReceiveMessages6/EPS_21A/CRC_Sub ==
  In1 : Inport
  Out1 : Outport
  wires:
  In1/1 -> Out1/1

== system VCU_CS75_9_30/长安CS75底盘程序，20ms一次/BSW_Input/DBC转化的messages（存底）/ReceiveMessages6/EPS_21A/EPS_AvailabilityStatus_Sub ==
  In1 : Inport
  Out1 : Outport
  wires:
  In1/1 -> Out1/1

== system VCU_CS75_9_30/长安CS75底盘程序，20ms一次/BSW_Input/DBC转化的messages（存底）/ReceiveMessages6/EPS_21A/EPS_IACC_abortReson_Sub ==
  In1 : Inport
  Out1 : Outport
  wires:
  In1/1 -> Out1/1

== system VCU_CS75_9_30/长安CS75底盘程序，20ms一次/BSW_Input/DBC转化的messages（存底）/ReceiveMessages6/EPS_21A/EPS_MeasTsionBatTorquevalid_Sub ==
  In1 : Inport
  Out1 : Outport
  wires:
  In1/1 -> Out1/1

== system VCU_CS75_9_30/长安CS75底盘程序，20ms一次/BSW_Input/DBC转化的messages（存底）/ReceiveMessages6/EPS_21A/EPS_MeasuredTosionBatTorque_Sub ==
  In1 : Inport
  Out1 : Outport
  wires:
  In1/1 -> Out1/1

== system VCU_CS75_9_30/长安CS75底盘程序，20ms一次/BSW_Input/DBC转化的messages（存底）/ReceiveMessages6/EPS_21A/Rollingcounter_Sub ==
  In1 : Inport
  Out1 : Outport
  wires:
  In1/1 -> Out1/1

== system VCU_CS75_9_30/长安CS75底盘程序，20ms一次/BSW_Input/DBC转化的messages（存底）/ReceiveMessages7/ESP_277/ESP_ABAactive_Sub ==
  In1 : Inport
  Out1 : Outport
  wires:
  In1/1 -> Out1/1

== system VCU_CS75_9_30/长安CS75底盘程序，20ms一次/BSW_Input/DBC转化的messages（存底）/ReceiveMessages7/ESP_277/ESP_ABAavailable_Sub ==
  In1 : Inport
  Out1 : Outport
  wires:
  In1/1 -> Out1/1

== system VCU_CS75_9_30/长安CS75底盘程序，20ms一次/BSW_Input/DBC转化的messages（存底）/ReceiveMessages7/ESP_277/ESP_AEBAvailable_Sub ==
  In1 : Inport
  Out1 : Outport
  wires:
  In1/1 -> Out1/1

== system VCU_CS75_9_30/长安CS75底盘程序，20ms一次/BSW_Input/DBC转化的messages（存底）/ReceiveMessages7/ESP_277/ESP_AEBdecActive_Sub ==
  In1 : Inport
  Out1 : Outport
  wires:
  In1/1 -> Out1/1

== system VCU_CS75_9_30/长安CS75底盘程序，20ms一次/BSW_Input/DBC转化的messages（存底）/ReceiveMessages7/ESP_277/ESP_AWBactive_Sub ==
  In1 : Inport
  Out1 : Outport
  wires:
  In1/1 -> Out1/1

== system VCU_CS75_9_30/长安CS75底盘程序，20ms一次/BSW_Input/DBC转化的messages（存底）/ReceiveMessages7/ESP_277/ESP_AWBavailable_Sub ==
  In1 : Inport
  Out1 : Outport
  wires:
  In1/1 -> Out1/1

== system VCU_CS75_9_30/长安CS75底盘程序，20ms一次/BSW_Input/DBC转化的messages（存底）/ReceiveMessages7/ESP_277/ESP_BrakeForce_Sub ==
  In1 : Inport
  Out1 : Outport
  wires:
  In1/1 -> Out1/1

== system VCU_CS75_9_30/长安CS75底盘程序，20ms一次/BSW_Input/DBC转化的messages（存底）/ReceiveMessages7/ESP_277/ESP_BrakeOverHeat_Sub ==
  In1 : Inport
  Out1 : Outport
  wires:
  In1/1 -> Out1/1

== system VCU_CS75_9_30/长安CS75底盘程序，20ms一次/BSW_Input/DBC转化的messages（存底）/ReceiveMessages7/ESP_277/ESP_CDD_Active_APA_Sub ==
  In1 : Inport
  Out1 : Outport
  wires:
  In1/1 -> Out1/1

== system VCU_CS75_9_30/长安CS75底盘程序，20ms一次/BSW_Input/DBC转化的messages（存底）/ReceiveMessages7/ESP_277/ESP_CDD_Active_Sub ==
  In1 : Inport
  Out1 : Outport
  wires:
  In1/1 -> Out1/1

== system VCU_CS75_9_30/长安CS75底盘程序，20ms一次/BSW_Input/DBC转化的messages（存底）/ReceiveMessages7/ESP_277/ESP_CDD_Available_APA_Sub ==
  In1 : Inport
  Out1 : Outport
  wires:
  In1/1 -> Out1/1

== system VCU_CS75_9_30/长安CS75底盘程序，20ms一次/BSW_Input/DBC转化的messages（存底）/ReceiveMessages7/ESP_277/ESP_CDD_Available_Sub ==
  In1 : Inport
  Out1 : Outport
  wires:
  In1/1 -> Out1/1

== system VCU_CS75_9_30/长安CS75底盘程序，20ms一次/BSW_Input/DBC转化的messages（存底）/ReceiveMessages7/ESP_277/ESP_CheckSum_277_Sub ==
  In1 : Inport
  Out1 : Outport
  wires:
  In1/1 -> Out1/1

== system VCU_CS75_9_30/长安CS75底盘程序，20ms一次/BSW_Input/DBC转化的messages（存底）/ReceiveMessages7/ESP_277/ESP_PrefillActive_Sub ==
  In1 : Inport
  Out1 : Outport
  wires:
  In1/1 -> Out1/1

== system VCU_CS75_9_30/长安CS75底盘程序，20ms一次/BSW_Input/DBC转化的messages（存底）/ReceiveMessages7/ESP_277/ESP_PrefillAvailable_Sub ==
  In1 : Inport
  Out1 : Outport
  wires:
  In1/1 -> Out1/1

== system VCU_CS75_9_30/长安CS75底盘程序，20ms一次/BSW_Input/DBC转化的messages（存底）/ReceiveMessages7/ESP_277/ESP_RollingCounter_277_Sub ==
  In1 : Inport
  Out1 : Outport
  wires:
  In1/1 -> Out1/1

== system VCU_CS75_9_30/长安CS75底盘程序，20ms一次/BSW_Input/DBC转化的messages（存底）/ReceiveMessages7/ESP_277/ESP_TCSActive_Sub ==
  In1 : Inport
  Out1 : Outport
  wires:
  In1/1 -> Out1/1

== system VCU_CS75_9_30/长安CS75底盘程序，20ms一次/BSW_Input/DBC转化的messages（存底）/ReceiveMessages7/ESP_277/ESP_VDCActive_Sub ==
  In1 : Inport
  Out1 : Outport
  wires:
  In1/1 -> Out1/1

== system VCU_CS75_9_30/长安CS75底盘程序，20ms一次/BSW_Input/DBC转化的messages（存底）/ReceiveMessages7/ESP_277/ESP_VehicleStandstill_Sub ==
  In1 : Inport
  Out1 : Outport
  wires:
  In1/1 -> Out1/1

== system VCU_CS75_9_30/长安CS75底盘程序，20ms一次/BSW_Input/DBC转化的messages（存底）/ReceiveMessages8/ESP_280/Wheel_Speed_FL_Data_Sub ==
  In1 : Inport
  Out1 : Outport
  wires:
  In1/1 -> Out1/1

== system VCU_CS75_9_30/长安CS75底盘程序，20ms一次/BSW_Input/DBC转化的messages（存底）/ReceiveMessages8/ESP_280/Wheel_Speed_FL_Direction_Sub ==
  In1 : Inport
  Out1 : Outport
  wires:
  In1/1 -> Out1/1

== system VCU_CS75_9_30/长安CS75底盘程序，20ms一次/BSW_Input/DBC转化的messages（存底）/ReceiveMessages8/ESP_280/Wheel_Speed_FL_Valid_Data_Sub ==
  In1 : Inport
  Out1 : Outport
  wires:
  In1/1 -> Out1/1

== system VCU_CS75_9_30/长安CS75底盘程序，20ms一次/BSW_Input/DBC转化的messages（存底）/ReceiveMessages8/ESP_280/Wheel_Speed_FR_Data_Sub ==
  In1 : Inport
  Out1 : Outport
  wires:
  In1/1 -> Out1/1

== system VCU_CS75_9_30/长安CS75底盘程序，20ms一次/BSW_Input/DBC转化的messages（存底）/ReceiveMessages8/ESP_280/Wheel_Speed_FR_Direction_Sub ==
  In1 : Inport
  Out1 : Outport
  wires:
  In1/1 -> Out1/1

== system VCU_CS75_9_30/长安CS75底盘程序，20ms一次/BSW_Input/DBC转化的messages（存底）/ReceiveMessages8/ESP_280/Wheel_Speed_FR_Valid_Data_Sub ==
  In1 : Inport
  Out1 : Outport
  wires:
  In1/1 -> Out1/1

== system VCU_CS75_9_30/长安CS75底盘程序，20ms一次/BSW_Input/DBC转化的messages（存底）/ReceiveMessages8/ESP_280/Wheel_Speed_RL_Data_Sub ==
  In1 : Inport
  Out1 : Outport
  wires:
  In1/1 -> Out1/1

== system VCU_CS75_9_30/长安CS75底盘程序，20ms一次/BSW_Input/DBC转化的messages（存底）/ReceiveMessages8/ESP_280/Wheel_Speed_RL_Direction_Sub ==
  In1 : Inport
  Out1 : Outport
  wires:
  In1/1 -> Out1/1

== system VCU_CS75_9_30/长安CS75底盘程序，20ms一次/BSW_Input/DBC转化的messages（存底）/ReceiveMessages8/ESP_280/Wheel_Speed_RL_Valid_Data_Sub ==
  In1 : Inport
  Out1 : Outport
  wires:
  In1/1 -> Out1/1

== system VCU_CS75_9_30/长安CS75底盘程序，20ms一次/BSW_Input/DBC转化的messages（存底）/ReceiveMessages8/ESP_280/Wheel_Speed_RR_Data_Sub ==
  In1 : Inport
  Out1 : Outport
  wires:
  In1/1 -> Out1/1

== system VCU_CS75_9_30/长安CS75底盘程序，20ms一次/BSW_Input/DBC转化的messages（存底）/ReceiveMessages8/ESP_280/Wheel_Speed_RR_Direction_Sub ==
  In1 : Inport
  Out1 : Outport
  wires:
  In1/1 -> Out1/1

== system VCU_CS75_9_30/长安CS75底盘程序，20ms一次/BSW_Input/DBC转化的messages（存底）/ReceiveMessages8/ESP_280/Wheel_Speed_RR_Valid_Data_Sub ==
  In1 : Inport
  Out1 : Outport
  wires:
  In1/1 -> Out1/1

== system VCU_CS75_9_30/长安CS75底盘程序，20ms一次/BSW_Input/DBC转化的messages（存底）/ReceiveMessages9/ESP_281/ESP_ABSActiveStatus_Sub ==
  In1 : Inport
  Out1 : Outport
  wires:
  In1/1 -> Out1/1

== system VCU_CS75_9_30/长安CS75底盘程序，20ms一次/BSW_Input/DBC转化的messages（存底）/ReceiveMessages9/ESP_281/ESP_ABSFailStatus_Sub ==
  In1 : Inport
  Out1 : Outport
  wires:
  In1/1 -> Out1/1

== system VCU_CS75_9_30/长安CS75底盘程序，20ms一次/BSW_Input/DBC转化的messages（存底）/ReceiveMessages9/ESP_281/ESP_BrakePedalStatus_Sub ==
  In1 : Inport
  Out1 : Outport
  wires:
  In1/1 -> Out1/1

== system VCU_CS75_9_30/长安CS75底盘程序，20ms一次/BSW_Input/DBC转化的messages（存底）/ReceiveMessages9/ESP_281/ESP_Checksum_Sub ==
  In1 : Inport
  Out1 : Outport
  wires:
  In1/1 -> Out1/1

== system VCU_CS75_9_30/长安CS75底盘程序，20ms一次/BSW_Input/DBC转化的messages（存底）/ReceiveMessages9/ESP_281/ESP_EBDFailStatus_Sub ==
  In1 : Inport
  Out1 : Outport
  wires:
  In1/1 -> Out1/1

== system VCU_CS75_9_30/长安CS75底盘程序，20ms一次/BSW_Input/DBC转化的messages（存底）/ReceiveMessages9/ESP_281/ESP_ESPActiveStatus_Sub ==
  In1 : Inport
  Out1 : Outport
  wires:
  In1/1 -> Out1/1

== system VCU_CS75_9_30/长安CS75底盘程序，20ms一次/BSW_Input/DBC转化的messages（存底）/ReceiveMessages9/ESP_281/ESP_ESPFailStatus_Sub ==
  In1 : Inport
  Out1 : Outport
  wires:
  In1/1 -> Out1/1

== system VCU_CS75_9_30/长安CS75底盘程序，20ms一次/BSW_Input/DBC转化的messages（存底）/ReceiveMessages9/ESP_281/ESP_ESPSwitchStatus_Sub ==
  In1 : Inport
  Out1 : Outport
  wires:
  In1/1 -> Out1/1

== system VCU_CS75_9_30/长安CS75底盘程序，20ms一次/BSW_Input/DBC转化的messages（存底）/ReceiveMessages9/ESP_281/ESP_RollingCounter_Sub ==
  In1 : Inport
  Out1 : Outport
  wires:
  In1/1 -> Out1/1

== system VCU_CS75_9_30/长安CS75底盘程序，20ms一次/BSW_Input/DBC转化的messages（存底）/ReceiveMessages9/ESP_281/ESP_VehicleSpeed_Status_Sub ==
  In1 : Inport
  Out1 : Outport
  wires:
  In1/1 -> Out1/1

== system VCU_CS75_9_30/长安CS75底盘程序，20ms一次/BSW_Input/DBC转化的messages（存底）/ReceiveMessages9/ESP_281/ESP_VehicleSpeed_Sub ==
  In1 : Inport
  Out1 : Outport
  wires:
  In1/1 -> Out1/1

== system VCU_CS75_9_30/长安CS75底盘程序，20ms一次/BSW_Output/CAN0_Tx/to511/VCU2IPC/Engine_Feedback ==
  Engine_Feedback : Inport
  Constant{1,3..8} (7 alike) : Constant  Value=0  OutDataTypeStr=uint8
  Engine_FeedbackRon : Rounding  Operator=round
  Engine_Feedback_1sat : Saturate  UpperLimit=255  LowerLimit=0
  Engine_Feedback_Convert : DataTypeConversion  OutDataTypeStr=uint8
  Engine_Feedback_Convert1 : DataTypeConversion  OutDataTypeStr=uint32
  Engine_Feedback_D : Product  Inputs=*/
  Engine_Feedback_F : Constant  Value=0.00784313725490196  OutDataTypeStr=single
  Engine_Feedback_L : simulink/Logic and Bit Operations/Bitwise Operator  logicop=AND  UseBitMask=on  BitMask=255  BitMaskRealWorld=Stored Integer
  Engine_Feedback_O : Constant  Value=-1  OutDataTypeStr=single
  Engine_Feedback_S : ArithShift
  Engine_Feedback_sat : Saturate  UpperLimit=1  LowerLimit=-1
  Engine_Feedback_st : Sum  Inputs=+-
  output1 : Outport
  output2 : Outport  Port=2
  output3 : Outport  Port=3
  output4 : Outport  Port=4
  output5 : Outport  Port=5
  output6 : Outport  Port=6
  output7 : Outport  Port=7
  output8 : Outport  Port=8
  wires:
  Engine_Feedback/1 -> Engine_Feedback_sat/1
  Engine_Feedback_sat/1 -> Engine_Feedback_st/1
  Engine_Feedback_O/1 -> Engine_Feedback_st/2
  Engine_Feedback_st/1 -> Engine_Feedback_D/1
  Engine_Feedback_F/1 -> Engine_Feedback_D/2
  Engine_Feedback_D/1 -> Engine_FeedbackRon/1
  Engine_FeedbackRon/1 -> Engine_Feedback_S/1
  Engine_Feedback_S/1 -> Engine_Feedback_1sat/1
  Engine_Feedback_1sat/1 -> Engine_Feedback_Convert1/1
  Engine_Feedback_Convert1/1 -> Engine_Feedback_L/1
  Engine_Feedback_L/1 -> Engine_Feedback_Convert/1
  Engine_Feedback_Convert/1 -> output2/1
  Constant1/1 -> output1/1
  Constant3/1 -> output3/1
  Constant4/1 -> output4/1
  Constant5/1 -> output5/1
  Constant6/1 -> output6/1
  Constant7/1 -> output7/1
  Constant8/1 -> output8/1

== system VCU_CS75_9_30/长安CS75底盘程序，20ms一次/BSW_Output/CAN0_Tx/to511/VCU2IPC/Engine_Feedback2 ==
  Engine_Feedback2 : Inport
  Constant{1..2,4..8} (7 alike) : Constant  Value=0  OutDataTypeStr=uint8
  Engine_Feedback2Ron : Rounding  Operator=round
  Engine_Feedback2_1sat : Saturate  UpperLimit=255  LowerLimit=0
  Engine_Feedback2_Convert : DataTypeConversion  OutDataTypeStr=uint8
  Engine_Feedback2_Convert1 : DataTypeConversion  OutDataTypeStr=uint32
  Engine_Feedback2_D : Product  Inputs=*/
  Engine_Feedback2_F : Constant  Value=0.00784313725490196  OutDataTypeStr=single
  Engine_Feedback2_L : simulink/Logic and Bit Operations/Bitwise Operator  logicop=AND  UseBitMask=on  BitMask=255  BitMaskRealWorld=Stored Integer
  Engine_Feedback2_O : Constant  Value=-1  OutDataTypeStr=single
  Engine_Feedback2_S : ArithShift
  Engine_Feedback2_sat : Saturate  UpperLimit=1  LowerLimit=-1
  Engine_Feedback2_st : Sum  Inputs=+-
  output1 : Outport
  output2 : Outport  Port=2
  output3 : Outport  Port=3
  output4 : Outport  Port=4
  output5 : Outport  Port=5
  output6 : Outport  Port=6
  output7 : Outport  Port=7
  output8 : Outport  Port=8
  wires:
  Engine_Feedback2/1 -> Engine_Feedback2_sat/1
  Engine_Feedback2_sat/1 -> Engine_Feedback2_st/1
  Engine_Feedback2_O/1 -> Engine_Feedback2_st/2
  Engine_Feedback2_st/1 -> Engine_Feedback2_D/1
  Engine_Feedback2_F/1 -> Engine_Feedback2_D/2
  Engine_Feedback2_D/1 -> Engine_Feedback2Ron/1
  Engine_Feedback2Ron/1 -> Engine_Feedback2_S/1
  Engine_Feedback2_S/1 -> Engine_Feedback2_1sat/1
  Engine_Feedback2_1sat/1 -> Engine_Feedback2_Convert1/1
  Engine_Feedback2_Convert1/1 -> Engine_Feedback2_L/1
  Engine_Feedback2_L/1 -> Engine_Feedback2_Convert/1
  Engine_Feedback2_Convert/1 -> output3/1
  Constant1/1 -> output1/1
  Constant2/1 -> output2/1
  Constant4/1 -> output4/1
  Constant5/1 -> output5/1
  Constant6/1 -> output6/1
  Constant7/1 -> output7/1
  Constant8/1 -> output8/1

== system VCU_CS75_9_30/长安CS75底盘程序，20ms一次/BSW_Output/CAN0_Tx/to511/VCU2IPC/Res_go ==
  Res_go : Inport
  Constant{1..5,7..8} (7 alike) : Constant  Value=0  OutDataTypeStr=uint8
  Res_goRon : Rounding  Operator=round
  Res_go_1sat : Saturate  UpperLimit=255  LowerLimit=0
  Res_go_Convert : DataTypeConversion  OutDataTypeStr=uint8
  Res_go_Convert1 : DataTypeConversion  OutDataTypeStr=uint32
  Res_go_D : Product  Inputs=*/
  Res_go_F : Constant  OutDataTypeStr=single
  Res_go_L : simulink/Logic and Bit Operations/Bitwise Operator  logicop=AND  UseBitMask=on  BitMask=255  BitMaskRealWorld=Stored Integer
  Res_go_O : Constant  Value=0  OutDataTypeStr=single
  Res_go_S : ArithShift
  Res_go_sat : Saturate  UpperLimit=1  LowerLimit=0
  Res_go_st : Sum  Inputs=+-
  output1 : Outport
  output2 : Outport  Port=2
  output3 : Outport  Port=3
  output4 : Outport  Port=4
  output5 : Outport  Port=5
  output6 : Outport  Port=6
  output7 : Outport  Port=7
  output8 : Outport  Port=8
  wires:
  Res_go/1 -> Res_go_sat/1
  Res_go_sat/1 -> Res_go_st/1
  Res_go_O/1 -> Res_go_st/2
  Res_go_st/1 -> Res_go_D/1
  Res_go_F/1 -> Res_go_D/2
  Res_go_D/1 -> Res_goRon/1
  Res_goRon/1 -> Res_go_S/1
  Res_go_S/1 -> Res_go_1sat/1
  Res_go_1sat/1 -> Res_go_Convert1/1
  Res_go_Convert1/1 -> Res_go_L/1
  Res_go_L/1 -> Res_go_Convert/1
  Res_go_Convert/1 -> output6/1
  Constant1/1 -> output1/1
  Constant2/1 -> output2/1
  Constant3/1 -> output3/1
  Constant4/1 -> output4/1
  Constant5/1 -> output5/1
  Constant7/1 -> output7/1
  Constant8/1 -> output8/1

== system VCU_CS75_9_30/长安CS75底盘程序，20ms一次/BSW_Output/CAN0_Tx/to511/VCU2IPC/Steering_Angle_Feedback ==
  Steering_Angle_Feedback : Inport
  Constant{2..8} (7 alike) : Constant  Value=0  OutDataTypeStr=uint8
  Steering_Angle_FeedbackRon : Rounding  Operator=round
  Steering_Angle_Feedback_1sat : Saturate  UpperLimit=255  LowerLimit=0
  Steering_Angle_Feedback_Convert : DataTypeConversion  OutDataTypeStr=uint8
  Steering_Angle_Feedback_Convert1 : DataTypeConversion  OutDataTypeStr=uint32
  Steering_Angle_Feedback_D : Product  Inputs=*/
  Steering_Angle_Feedback_F : Constant  Value=0.005474  OutDataTypeStr=single
  Steering_Angle_Feedback_L : simulink/Logic and Bit Operations/Bitwise Operator  logicop=AND  UseBitMask=on  BitMask=255  BitMaskRealWorld=Stored Integer
  Steering_Angle_Feedback_O : Constant  Value=-0.698  OutDataTypeStr=single
  Steering_Angle_Feedback_S : ArithShift
  Steering_Angle_Feedback_sat : Saturate  UpperLimit=0.69787  LowerLimit=-0.698
  Steering_Angle_Feedback_st : Sum  Inputs=+-
  output1 : Outport
  output2 : Outport  Port=2
  output3 : Outport  Port=3
  output4 : Outport  Port=4
  output5 : Outport  Port=5
  output6 : Outport  Port=6
  output7 : Outport  Port=7
  output8 : Outport  Port=8
  wires:
  Steering_Angle_Feedback/1 -> Steering_Angle_Feedback_sat/1
  Steering_Angle_Feedback_sat/1 -> Steering_Angle_Feedback_st/1
  Steering_Angle_Feedback_O/1 -> Steering_Angle_Feedback_st/2
  Steering_Angle_Feedback_st/1 -> Steering_Angle_Feedback_D/1
  Steering_Angle_Feedback_F/1 -> Steering_Angle_Feedback_D/2
  Steering_Angle_Feedback_D/1 -> Steering_Angle_FeedbackRon/1
  Steering_Angle_FeedbackRon/1 -> Steering_Angle_Feedback_S/1
  Steering_Angle_Feedback_S/1 -> Steering_Angle_Feedback_1sat/1
  Steering_Angle_Feedback_1sat/1 -> Steering_Angle_Feedback_Convert1/1
  Steering_Angle_Feedback_Convert1/1 -> Steering_Angle_Feedback_L/1
  Steering_Angle_Feedback_L/1 -> Steering_Angle_Feedback_Convert/1
  Steering_Angle_Feedback_Convert/1 -> output1/1
  Constant2/1 -> output2/1
  Constant3/1 -> output3/1
  Constant4/1 -> output4/1
  Constant5/1 -> output5/1
  Constant6/1 -> output6/1
  Constant7/1 -> output7/1
  Constant8/1 -> output8/1

== system VCU_CS75_9_30/长安CS75底盘程序，20ms一次/BSW_Output/CAN0_Tx/to511/VCU2IPC/Steering_feedback ==
  Steering_feedback : Inport
  BitCov : DataTypeConversion  OutDataTypeStr=uint8
  Constant{1..6} (6 alike) : Constant  Value=0  OutDataTypeStr=uint8
  Steering_feedbackCOV : DataTypeConversion  OutDataTypeStr=uint8
  Steering_feedbackRon : Rounding  Operator=round
  Steering_feedback_1sat : Saturate  UpperLimit=65535  LowerLimit=0
  Steering_feedback_And : simulink/Logic and Bit Operations/Bitwise Operator  logicop=AND  UseBitMask=off  NumInputPorts=2  BitMask=bin2dec('11011001')  BitMaskRealWorld=Stored Integer
  Steering_feedback_And_C : Constant  Value=255  OutDataTypeStr=uint32
  Steering_feedback_Convert : DataTypeConversion  OutDataTypeStr=uint32
  Steering_feedback_D : Product  Inputs=*/
  Steering_feedback_D1 : Product  Inputs=*/
  Steering_feedback_F : Constant  Value=0.015259  OutDataTypeStr=single
  Steering_feedback_L : simulink/Logic and Bit Operations/Bitwise Operator  logicop=AND  UseBitMask=on  BitMask=65535  BitMaskRealWorld=Stored Integer
  Steering_feedback_O : Constant  Value=-500  OutDataTypeStr=single
  Steering_feedback_S : ArithShift
  Steering_feedback_sat : Saturate  UpperLimit=499.998565  LowerLimit=-500
  Steering_feedback_st : Sum  Inputs=+-
  Steering_feedbackoutput8_C : Constant  Value=256
  output1 : Outport
  output2 : Outport  Port=2
  output3 : Outport  Port=3
  output4 : Outport  Port=4
  output5 : Outport  Port=5
  output6 : Outport  Port=6
  output7 : Outport  Port=7
  output8 : Outport  Port=8
  wires:
  Steering_feedback/1 -> Steering_feedback_sat/1
  Steering_feedback_sat/1 -> Steering_feedback_st/1
  Steering_feedback_O/1 -> Steering_feedback_st/2
  Steering_feedback_st/1 -> Steering_feedback_D/1
  Steering_feedback_F/1 -> Steering_feedback_D/2
  Steering_feedback_D/1 -> Steering_feedbackRon/1
  Steering_feedbackRon/1 -> Steering_feedback_S/1
  Steering_feedback_S/1 -> Steering_feedback_1sat/1
  Steering_feedback_1sat/1 -> Steering_feedback_Convert/1
  Steering_feedback_Convert/1 -> Steering_feedback_L/1
  Steering_feedback_L/1 -> Steering_feedback_D1/1, Steering_feedback_And/1
  Steering_feedbackoutput8_C/1 -> Steering_feedback_D1/2
  Steering_feedback_D1/1 -> Steering_feedbackCOV/1
  Steering_feedbackCOV/1 -> output8/1
  Steering_feedback_And_C/1 -> Steering_feedback_And/2
  Steering_feedback_And/1 -> BitCov/1
  BitCov/1 -> output7/1
  Constant1/1 -> output1/1
  Constant2/1 -> output2/1
  Constant3/1 -> output3/1
  Constant4/1 -> output4/1
  Constant5/1 -> output5/1
  Constant6/1 -> output6/1

== system VCU_CS75_9_30/长安CS75底盘程序，20ms一次/BSW_Output/CAN0_Tx/to511/VCU2IPC/Wheel_Speed_RL_Feedback ==
  Wheel_Speed_RL_Feedback : Inport
  Constant{1..3,5..8} (7 alike) : Constant  Value=0  OutDataTypeStr=uint8
  Wheel_Speed_RL_FeedbackRon : Rounding  Operator=round
  Wheel_Speed_RL_Feedback_1sat : Saturate  UpperLimit=255  LowerLimit=0
  Wheel_Speed_RL_Feedback_Convert : DataTypeConversion  OutDataTypeStr=uint8
  Wheel_Speed_RL_Feedback_Convert1 : DataTypeConversion  OutDataTypeStr=uint32
  Wheel_Speed_RL_Feedback_D : Product  Inputs=*/
  Wheel_Speed_RL_Feedback_F : Constant  Value=0.784313725490196  OutDataTypeStr=single
  Wheel_Speed_RL_Feedback_L : simulink/Logic and Bit Operations/Bitwise Operator  logicop=AND  UseBitMask=on  BitMask=255  BitMaskRealWorld=Stored Integer
  Wheel_Speed_RL_Feedback_O : Constant  Value=0  OutDataTypeStr=single
  Wheel_Speed_RL_Feedback_S : ArithShift
  Wheel_Speed_RL_Feedback_sat : Saturate  UpperLimit=200  LowerLimit=0
  Wheel_Speed_RL_Feedback_st : Sum  Inputs=+-
  output1 : Outport
  output2 : Outport  Port=2
  output3 : Outport  Port=3
  output4 : Outport  Port=4
  output5 : Outport  Port=5
  output6 : Outport  Port=6
  output7 : Outport  Port=7
  output8 : Outport  Port=8
  wires:
  Wheel_Speed_RL_Feedback/1 -> Wheel_Speed_RL_Feedback_sat/1
  Wheel_Speed_RL_Feedback_sat/1 -> Wheel_Speed_RL_Feedback_st/1
  Wheel_Speed_RL_Feedback_O/1 -> Wheel_Speed_RL_Feedback_st/2
  Wheel_Speed_RL_Feedback_st/1 -> Wheel_Speed_RL_Feedback_D/1
  Wheel_Speed_RL_Feedback_F/1 -> Wheel_Speed_RL_Feedback_D/2
  Wheel_Speed_RL_Feedback_D/1 -> Wheel_Speed_RL_FeedbackRon/1
  Wheel_Speed_RL_FeedbackRon/1 -> Wheel_Speed_RL_Feedback_S/1
  Wheel_Speed_RL_Feedback_S/1 -> Wheel_Speed_RL_Feedback_1sat/1
  Wheel_Speed_RL_Feedback_1sat/1 -> Wheel_Speed_RL_Feedback_Convert1/1
  Wheel_Speed_RL_Feedback_Convert1/1 -> Wheel_Speed_RL_Feedback_L/1
  Wheel_Speed_RL_Feedback_L/1 -> Wheel_Speed_RL_Feedback_Convert/1
  Wheel_Speed_RL_Feedback_Convert/1 -> output4/1
  Constant1/1 -> output1/1
  Constant2/1 -> output2/1
  Constant3/1 -> output3/1
  Constant5/1 -> output5/1
  Constant6/1 -> output6/1
  Constant7/1 -> output7/1
  Constant8/1 -> output8/1
